simulink model "mpc_active_suspension"  (R2023a)
settings: Solver=VariableStepAuto  StartTime=0.0  StopTime=10.0  RelTol=1e-3
values from neighbouring files (symbols this model uses):
  A = [0, 1, 0, -1 ... (first row only)    [setup_model.m]
  B_full = [Bu, Bmd]    [setup_model.m]
  C = [-ks/ms, -cs/ms, 0, cs/ms ... (first row only)    [setup_model.m]
  cs = 1000    [setup_model.m]
  D_full = [Du, Dmd]    [setup_model.m]
  ks = 16812    [setup_model.m]
  kt = 190000    [setup_model.m]
  ms = 290    [setup_model.m]
  mus = 60    [setup_model.m]
libraries: mpclib x1
settings Model: Creator=Adham  LastModifiedBy=Adham

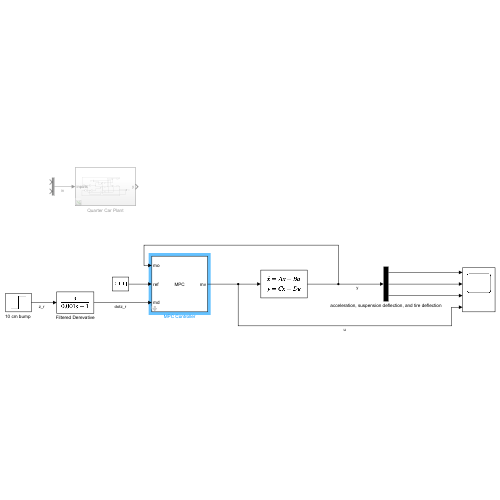
[thumbnail: Simulink's stored preview of the top-level diagram]
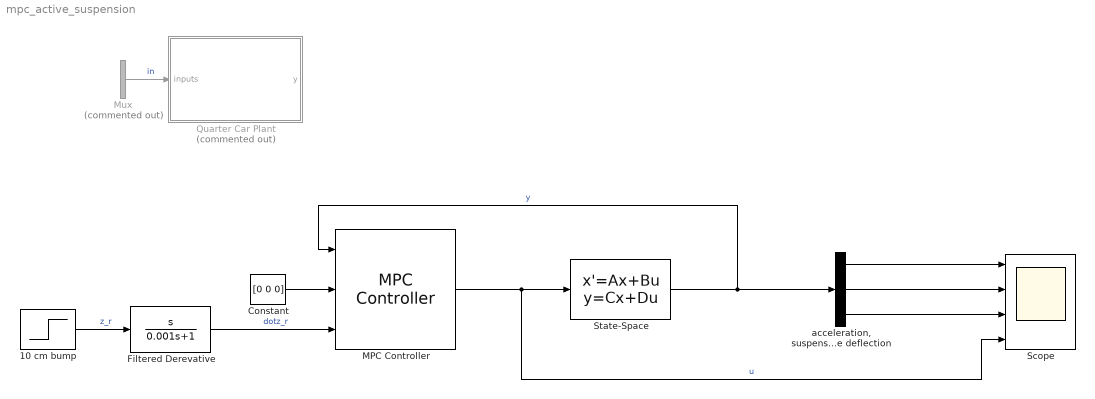
== system mpc_active_suspension ==
  "10 cm bump " : Step  After=0.1  SampleTime=0
  Constant : Constant  Value=[0 0 0]
  Filtered Derevative : TransferFcn  Numerator=[1 0]  Denominator=[0.001 1]
  MPC Controller : mpclib/MPC Controller  SCDEnableBlockLinearizationSpecification=on  is_multiple=0  enable_value=0  return_u0=off  updateMPCinCallerWorkspace=on  md_inport=on  mv_inport=off  uref_inport=off  return_cost=off  return_mvseq=off  return_qpstatus=off  return_xseq=off  return_state=off  return_ovseq=off  state_inport=off  umin_inport=off  umax_inport=off  ymin_inport=off  ymax_inport=off  cc_inport=off  ywt_inport=off  uwt_inport=off  duwt_inport=off  rhoeps_inport=off  pm_inport=off  MaximumP=10  HorizonChoice=FixedHorizon  n_ts=0.01  n_p=10  n_mv=1  n_md=1  n_ud=0  n_mo=3  n_uo=0  BlockDataType=double  SampleTimeInherited=off  switch_inport=off
  Mux : Mux  Commented=on  Inputs=2
  Quarter Car Plant : Subsystem  Commented=on
  Scope : Scope  NumInputPorts=4
  State-Space : StateSpace  A=A  B=B_full  C=C  D=D_full  InitialCondition=0
  "acceleration, suspension deflection, and tire deflection" : Demux  Outputs=3
  wires:
  MPC Controller/1 -> State-Space/1, Scope/4  "u"
  "10 cm bump "/1 -> Filtered Derevative/1  "z_r"
  Filtered Derevative/1 -> MPC Controller/3  "dotz_r"
  "acceleration, suspension deflection, and tire deflection"/1 -> Scope/1
  "acceleration, suspension deflection, and tire deflection"/2 -> Scope/2
  "acceleration, suspension deflection, and tire deflection"/3 -> Scope/3
  Mux/1 -> Quarter Car Plant/1(inputs)  "in"
  Constant/1 -> MPC Controller/2
  State-Space/1 -> MPC Controller/1, "acceleration, suspension deflection, and tire deflection"/1  "y"

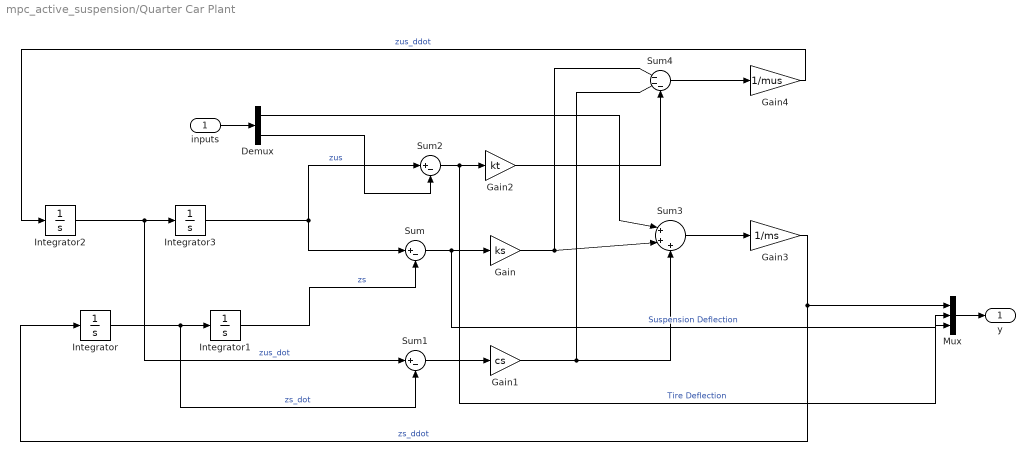
== system mpc_active_suspension/Quarter Car Plant ==
  inputs : Inport
  Demux : Demux  Outputs=2
  Gain : Gain  Gain=ks
  Gain1 : Gain  Gain=cs
  Gain2 : Gain  Gain=kt
  Gain3 : Gain  Gain=1/ms
  Gain4 : Gain  Gain=1/mus
  Integrator{,1..3} (4 alike) : Integrator
  Mux : Mux  Inputs=3
  Sum : Sum  Inputs=|+-
  Sum1 : Sum  Inputs=|+-
  Sum2 : Sum  Inputs=|+-
  Sum3 : Sum  Inputs=|+++
  Sum4 : Sum  Inputs=|---
  y : Outport
  wires:
  Integrator/1 -> Sum1/2, Integrator1/1  "zs_dot"
  Integrator1/1 -> Sum/2  "zs"
  Integrator2/1 -> Sum1/1, Integrator3/1  "zus_dot"
  Integrator3/1 -> Sum/1, Sum2/1  "zus"
  Gain3/1 -> Mux/1, Integrator/1  "zs_ddot"
  Gain4/1 -> Integrator2/1  "zus_ddot"
  Sum/1 -> Mux/2, Gain/1  "Suspension Deflection"
  Sum1/1 -> Gain1/1
  Demux/2 -> Sum2/2
  Sum2/1 -> Mux/3, Gain2/1  "Tire Deflection"
  Gain/1 -> Sum4/1, Sum3/2
  Gain1/1 -> Sum4/2, Sum3/3
  Sum3/1 -> Gain3/1
  Gain2/1 -> Sum4/3
  Sum4/1 -> Gain4/1
  Mux/1 -> y/1
  inputs/1 -> Demux/1
  Demux/1 -> Sum3/1
